simulink model "Experiment_Qcar_Dual_Mode_FL_MPC"  (R2022b)
settings: Solver=ode2  StartTime=0.0  StopTime=Tf  FixedStep=Ts2  RelTol=1e-3  EnableMultiTasking=on
values from neighbouring files (symbols this model uses):
  alpha_kalman = 0.9    [setup_FL_MPC.m]    (also in setup_NL_MPC.m; setup_backstepping.m)
  beta_kalman = 2    [setup_FL_MPC.m]    (also in setup_NL_MPC.m; setup_backstepping.m)
  Delta = 0.35    [setup_FL_MPC.m]
  g_N = P_N.b    [setup_FL_MPC.m]
  H_N = P_N.A    [setup_FL_MPC.m]
  H_w = H_w/g_w(1)    [setup_FL_MPC.m]
  K = 5*eye(2)    [setup_FL_MPC.m]
  kappa_kalman = 0    [setup_FL_MPC.m]    (also in setup_NL_MPC.m; setup_backstepping.m)
  l = 0.256    [setup_FL_MPC.m]    (also in setup_NL_MPC.m; setup_backstepping.m)
  Linv = linsolve(L,eye(size(L)),struct('LT',true))    [setup_FL_MPC.m]
  N = 10    [setup_FL_MPC.m]    (also in setup_NL_MPC.m; setup_backstepping.m = 5)
  P0_kalman = diag([1e-5 1e-5 1e-6 1e-6])    [setup_FL_MPC.m]    (also in setup_NL_MPC.m; setup_backstepping.m)
  q0 = [x0;y0;theta0;0]    [setup_FL_MPC.m]    (also in setup_NL_MPC.m; setup_backstepping.m)
  Q_kalman = diag([0.001 0.001 0.1 1])    [setup_FL_MPC.m]    (also in setup_NL_MPC.m = diag([0.001 0.001 0.1 10]); setup_backstepping.m = diag([0.001 0.001 0.1 10]))
  qu = 0.01    [setup_FL_MPC.m]    (also in setup_NL_MPC.m = 0.002)
  qz = 1    [setup_FL_MPC.m]    (also in setup_NL_MPC.m)
  R_kalman = diag([2e-5 2e-5 0.0001 0.001])    [setup_FL_MPC.m]    (also in setup_NL_MPC.m = diag([2e-5 2e-5 0.0001 0.00001]); setup_backstepping.m = diag([2e-5 2e-5 0.0001 0.00001]))
  theta0 = vicon_data(6)    [setup_FL_MPC.m]    (also in setup_NL_MPC.m; setup_backstepping.m)
  Ts = 0.008    [setup_FL_MPC.m]    (also in setup_NL_MPC.m = 0.01; setup_backstepping.m = 0.01)
  Ts2 = Ts    (= 0.008)    [setup_FL_MPC.m]    (also in setup_NL_MPC.m = 0.01; setup_backstepping.m = 0.01)
  v1max = 1    [setup_FL_MPC.m]    (also in setup_NL_MPC.m; setup_backstepping.m)
  v2max = 10    [setup_FL_MPC.m]    (also in setup_NL_MPC.m; setup_backstepping.m)
  x0 = vicon_data(1)    [setup_FL_MPC.m]    (also in setup_NL_MPC.m; setup_backstepping.m)
  y0 = vicon_data(2)    [setup_FL_MPC.m]    (also in setup_NL_MPC.m; setup_backstepping.m)
undefined symbols (not defined in the file or in its folder): DiscIntNeverNeededParam, HIL
libraries: quarc_library x17, simulink x2, dspsigops x1, slpidlib x1
(part 2 of 2)

== matlab function Experiment_Qcar_Dual_Mode_FL_MPC/Controller/MPC_active_set_nonconservative ==
  data: q input; v output; qr input; vr input; l input; Delta input; N input; Ts input; v1max input; v2max input; H_w input
function v = MPC_active_set_worst_case(q,qr,vr,l,Delta,N,Ts,v1max,v2max,H_w)


qz=1; qu=0.01;


x=q(1); y=q(2); theta=q(3); phi=q(4);

%Feedback linearized system state
z_k=[x+l*cos(theta)+Delta*cos(phi+theta);
    y+l*sin(theta)+Delta*sin(phi+theta)];


Wr=zeros(2*N,1);
R=zeros(2*N,1);



for i=1:N
    xr=qr(1,i); yr=qr(2,i); thetar=qr(3,i); phir=qr(4,i);
    v1r=vr(1,i); v2r=vr(2,i);

    %Feedback linearized system reference at time k+i
    zr_k=[xr+l*cos(thetar)+Delta*cos(phir+thetar);
        yr+l*sin(thetar)+Delta*sin(phir+thetar)];

    R(2*i-1:2*i,1)=zr_k;

    %Feedback Linearization reference transformation
    T_FL_r=[cos(thetar)-tan(phir)*(sin(thetar)+Delta*sin(thetar+phir)/l) -Delta*sin(thetar+phir);
        sin(thetar)+tan(phir)*(cos(thetar)+Delta*cos(thetar+phir)/l) Delta*cos(thetar+phir)];

    ur_k=T_FL_r*[v1r;v2r];

    Wr(2*i-1:2*i,1)=ur_k;


end


%Feedback Linearization state transformation
T_FL=[cos(theta)-tan(phi)*(sin(theta)+Delta*sin(theta+phi)/l) -Delta*sin(theta+phi);
    sin(theta)+tan(phi)*(cos(theta)+Delta*cos(theta+phi)/l) Delta*cos(theta+phi)];





Phi=repmat(eye(2),N,1);
Theta=Ts*repmat(eye(2),N);
Theta=tril(Theta);
Qhat=qz*eye(2*N);
Rhat=qu*eye(2*N);







H_obj=Theta'*Qhat*Theta+Rhat;
f_obj=Theta'*Qhat*Phi*z_k-Theta'*Qhat*Theta*Wr-Theta'*Qhat*R;

T=[-1 0; 0 -1; 1 0; 0 1];
Hk=T/T_FL;
g=[v1max;v2max;v1max;v2max];

H_constr=zeros(4,2*N);
H_constr(1:4,1:2)=Hk;

% for i=1:N-1
%     
%     H_constr(4+(i-1)*Nc+1:4+(i-1)*Nc+Nc,2*i+1:2*i+2)=H_w;
% 
% 
% end



g_constr=zeros(size(H_constr,1),1);
g_constr(1:4)=g;




% options = optimoptions('quadprog','Algorithm','active-set');
% usol =  quadprog(H_obj,f_obj,H_constr,g_constr,[],[],[],[],zeros(2*N,1),options);




% opt.MaxIterations = 100;
% opt.ConstraintTolerance = 1.0e-6;
% opt.OptimalityTolerance = 1.0e-6;

opt = mpcInteriorPointOptions;
% usol=mpcInteriorPointSolver(H_obj,f_obj,H_constr,g_constr,zeros(0,2*N),zeros(0,1),zeros(2*N,1),opt);


opt.UseHessianAsInput = true;
iA0 = false(size(g_constr));
usol=mpcActiveSetSolver(H_obj,f_obj,H_constr,g_constr,zeros(0,2*N),zeros(0,1),iA0,opt);



uk=usol(1:2);



v=T_FL\uk;

== matlab function Experiment_Qcar_Dual_Mode_FL_MPC/Controller/MPC_active_set2 ==
  data: q input; v output; qr input; vr input; l input; Delta input; N input; Ts input; v1max input; v2max input; H_w input
function v = MPC_active_set_worst_case(q,qr,vr,l,Delta,N,Ts,v1max,v2max,H_w)


qz=1; qu=0.01;


x=q(1); y=q(2); theta=q(3); phi=q(4);

%Feedback linearized system state
z_k=[x+l*cos(theta)+Delta*cos(phi+theta);
    y+l*sin(theta)+Delta*sin(phi+theta)];


Wr=zeros(2*N,1);
R=zeros(2*N,1);



for i=1:N
    xr=qr(1,i); yr=qr(2,i); thetar=qr(3,i); phir=qr(4,i);
    v1r=vr(1,i); v2r=vr(2,i);

    %Feedback linearized system reference at time k+i
    zr_k=[xr+l*cos(thetar)+Delta*cos(phir+thetar);
        yr+l*sin(thetar)+Delta*sin(phir+thetar)];

    R(2*i-1:2*i,1)=zr_k;

    %Feedback Linearization reference transformation
    T_FL_r=[cos(thetar)-tan(phir)*(sin(thetar)+Delta*sin(thetar+phir)/l) -Delta*sin(thetar+phir);
        sin(thetar)+tan(phir)*(cos(thetar)+Delta*cos(thetar+phir)/l) Delta*cos(thetar+phir)];

    ur_k=T_FL_r*[v1r;v2r];

    Wr(2*i-1:2*i,1)=ur_k;


end


%Feedback Linearization state transformation
T_FL=[cos(theta)-tan(phi)*(sin(theta)+Delta*sin(theta+phi)/l) -Delta*sin(theta+phi);
    sin(theta)+tan(phi)*(cos(theta)+Delta*cos(theta+phi)/l) Delta*cos(theta+phi)];





Phi=repmat(eye(2),N,1);
Theta=Ts*repmat(eye(2),N);
Theta=tril(Theta);
Qhat=qz*eye(2*N);
Rhat=qu*eye(2*N);







H_obj=Theta'*Qhat*Theta+Rhat;
f_obj=Theta'*Qhat*Phi*z_k-Theta'*Qhat*Theta*Wr-Theta'*Qhat*R;

T=[-1 0; 0 -1; 1 0; 0 1];
Hk=T/T_FL;
g=[v1max;v2max;v1max;v2max];


Nc=size(H_w,1);
H_constr=zeros(4+Nc*(N-1),2*N);
H_constr(1:4,1:2)=Hk;

for i=1:N-1
    
    H_constr(4+(i-1)*Nc+1:4+(i-1)*Nc+Nc,2*i+1:2*i+2)=H_w;


end



g_constr=ones(size(H_constr,1),1);
g_constr(1:4)=g;




% options = optimoptions('quadprog','Algorithm','active-set');
% usol =  quadprog(H_obj,f_obj,H_constr,g_constr,[],[],[],[],zeros(2*N,1),options);




% opt.MaxIterations = 100;
% opt.ConstraintTolerance = 1.0e-6;
% opt.OptimalityTolerance = 1.0e-6;

opt = mpcInteriorPointOptions;
% usol=mpcInteriorPointSolver(H_obj,f_obj,H_constr,g_constr,zeros(0,2*N),zeros(0,1),zeros(2*N,1),opt);
opt.UseHessianAsInput = true;
iA0 = false(size(g_constr));
usol=mpcActiveSetSolver(H_obj,f_obj,H_constr,g_constr,zeros(0,2*N),zeros(0,1),iA0,opt);



uk=usol(1:2);



v=T_FL\uk;

== matlab function Experiment_Qcar_Dual_Mode_FL_MPC/Controller/MPC_active_set ==
  data: q input; v output; qr input; vr input; l input; Delta input; N input; Ts input; v1max input; v2max input; H_w input
function v = MPC_active_set_worst_case(q,qr,vr,l,Delta,N,Ts,v1max,v2max,H_w)


qz=1; qu=0.01;


x=q(1); y=q(2); theta=q(3); phi=q(4);

%Feedback linearized system state
z_k=[x+l*cos(theta)+Delta*cos(phi+theta);
    y+l*sin(theta)+Delta*sin(phi+theta)];


Wr=zeros(2*N,1);
R=zeros(2*N,1);



for i=1:N
    xr=qr(1,i); yr=qr(2,i); thetar=qr(3,i); phir=qr(4,i);
    v1r=vr(1,i); v2r=vr(2,i);

    %Feedback linearized system reference at time k+i
    zr_k=[xr+l*cos(thetar)+Delta*cos(phir+thetar);
        yr+l*sin(thetar)+Delta*sin(phir+thetar)];

    R(2*i-1:2*i,1)=zr_k;

    %Feedback Linearization reference transformation
    T_FL_r=[cos(thetar)-tan(phir)*(sin(thetar)+Delta*sin(thetar+phir)/l) -Delta*sin(thetar+phir);
        sin(thetar)+tan(phir)*(cos(thetar)+Delta*cos(thetar+phir)/l) Delta*cos(thetar+phir)];

    ur_k=T_FL_r*[v1r;v2r];

    Wr(2*i-1:2*i,1)=ur_k;


end


%Feedback Linearization state transformation
T_FL=[cos(theta)-tan(phi)*(sin(theta)+Delta*sin(theta+phi)/l) -Delta*sin(theta+phi);
    sin(theta)+tan(phi)*(cos(theta)+Delta*cos(theta+phi)/l) Delta*cos(theta+phi)];





Phi=repmat(eye(2),N,1);
Theta=Ts*repmat(eye(2),N);
Theta=tril(Theta);
Qhat=qz*eye(2*N);
Rhat=qu*eye(2*N);







H_obj=Theta'*Qhat*Theta+Rhat;
f_obj=Theta'*Qhat*Phi*z_k-Theta'*Qhat*Theta*Wr-Theta'*Qhat*R;

T=[-1 0; 0 -1; 1 0; 0 1];
Hk=T/T_FL;
g=[v1max;v2max;v1max;v2max];


Nc=size(H_w,1);
H_constr=zeros(4+Nc*(N-1),2*N);
H_constr(1:4,1:2)=Hk;

% for i=1:N-1
%     
%     H_constr(4+(i-1)*Nc+1:4+(i-1)*Nc+Nc,2*i+1:2*i+2)=H_w;
% 
% 
% end



g_constr=zeros(size(H_constr,1),1);
g_constr(1:4)=g;




% options = optimoptions('quadprog','Algorithm','active-set');
% usol =  quadprog(H_obj,f_obj,H_constr,g_constr,[],[],[],[],zeros(2*N,1),options);




% opt.MaxIterations = 100;
% opt.ConstraintTolerance = 1.0e-6;
% opt.OptimalityTolerance = 1.0e-6;

opt = mpcInteriorPointOptions;
% usol=mpcInteriorPointSolver(H_obj,f_obj,H_constr,g_constr,zeros(0,2*N),zeros(0,1),zeros(2*N,1),opt);


opt.UseHessianAsInput = true;
iA0 = false(size(g_constr));
usol=mpcActiveSetSolver(H_obj,f_obj,H_constr,g_constr,zeros(0,2*N),zeros(0,1),iA0,opt);



uk=usol(1:2);



v=T_FL\uk;

== matlab function Experiment_Qcar_Dual_Mode_FL_MPC/Controller/MPC_interior_point_polyhedral_approx ==
  data: q input; v output; qr input; vr input; l input; Delta input; N input; Ts input; v1max input; v2max input; H_w input; qz input; qu input
function v = MPC_interior_point_polyhedral_approx(q,qr,vr,l,Delta,N,Ts,v1max,v2max,H_w,qz,qu)


x=q(1); y=q(2); theta=q(3); phi=q(4);

%Feedback linearized system state
z_k=[x+l*cos(theta)+Delta*cos(phi+theta);
     y+l*sin(theta)+Delta*sin(phi+theta)];


xr=qr(1,1); yr=qr(2,1); thetar=qr(3,1); phir=qr(4,1);
%Feedback linearized system reference at time k+i
zr_k=[xr+l*cos(thetar)+Delta*cos(phir+thetar);
      yr+l*sin(thetar)+Delta*sin(phir+thetar)];

ztilde_k=z_k-zr_k;


Wr=zeros(2*N,1);
% R=zeros(2*N,1);



for i=1:N
    thetar=qr(3,i); phir=qr(4,i);
    v1r=vr(1,i); v2r=vr(2,i);

    %     R(2*i-1:2*i,1)=zr_k;

    %Feedback Linearization reference transformation
    T_FL_r=[cos(thetar)-tan(phir)*(sin(thetar)+Delta*sin(thetar+phir)/l) -Delta*sin(thetar+phir);
        sin(thetar)+tan(phir)*(cos(thetar)+Delta*cos(thetar+phir)/l) Delta*cos(thetar+phir)];

    ur_k=T_FL_r*[v1r;v2r];

    Wr(2*i-1:2*i,1)=ur_k;


end


%Feedback Linearization state transformation
T_FL=[cos(theta)-tan(phi)*(sin(theta)+Delta*sin(theta+phi)/l) -Delta*sin(theta+phi);
    sin(theta)+tan(phi)*(cos(theta)+Delta*cos(theta+phi)/l) Delta*cos(theta+phi)];





Phi=repmat(eye(2),N,1);
Theta=Ts*repmat(eye(2),N);
Theta=tril(Theta);
Qhat=qz*eye(2*N);
Rhat=qu*eye(2*N);





H_obj=Theta'*Qhat*Theta+Rhat;
f_obj=Theta'*Qhat*Phi*ztilde_k-Theta'*Qhat*Theta*Wr-Rhat*Wr;

T=[-1 0; 0 -1; 1 0; 0 1];
Hk=T/T_FL;
g=[v1max;v2max;v1max;v2max];



Nc=size(H_w,1);
H_constr=zeros(4+Nc*(N-1),2*N);
H_constr(1:4,1:2)=Hk;

for i=1:N-1
    
    H_constr(4+(i-1)*Nc+1:4+(i-1)*Nc+Nc,2*i+1:2*i+2)=H_w;


end

g_constr=ones(size(H_constr,1),1);
g_constr(1:4)=g;



% options = optimoptions('quadprog','Algorithm','active-set');
% usol =  quadprog(H_obj,f_obj,H_constr,g_constr,[],[],[],[],zeros(2*N,1),options);




opt = mpcInteriorPointOptions;

opt.MaxIterations = 100;
opt.ConstraintTolerance = 1.0e-6;
opt.OptimalityTolerance = 1.0e-6;

usol=mpcInteriorPointSolver(H_obj,f_obj,H_constr,g_constr,zeros(0,2*N),zeros(0,1),zeros(2*N,1),opt);

%
% opt.UseHessianAsInput = true;
% iA0 = false(size(g_constr));
% usol=mpcActiveSetSolver(H_obj,f_obj,H_constr,g_constr,zeros(0,2*N),zeros(0,1),iA0,opt);
%


uk=usol(1:2);



v=T_FL\uk;
